simulink model "bObserver"  (R2020a)
settings: Solver=VariableStepAuto  StartTime=0.0  StopTime=1.5  FixedStep=0.0005  EnableMultiTasking=on
InitFcn:
  | kp=0.01;
  | ki=0.01;
  | 
  | k=2;
  | em=100000000;
  | GE=1/em;
  | GU=k*ki/GE;
  | GCE=k*kp/GU;
model workspace (MAT data in the model file):
  time = 0.8
values from neighbouring files (symbols this model uses):
  A1 = obj.boostConverter.A1    [BoostController.m]    (also in BoostConverter.m = [-obj.R/obj.L 0;0 -1/(obj.Ro*obj.C)]; BuckBoostConverter.m = [-obj.R/obj.L 0;0 -1/(obj.Ro*obj.C)]; obsmc.m = Asigma{1,1}; workspace_atual.mat = [-16.4  0; 0  -3.50877192982])
  A2 = obj.boostConverter.A2    [BoostController.m]    (also in BoostConverter.m = [-obj.R/obj.L -1/obj.L;1/obj.C -1/(obj.Ro*obj.C)]; BuckBoostConverter.m = [-obj.R/obj.L 1/obj.L;-1/obj.C -1/(obj.Ro*obj.C)]; obsmc.m = Asigma{1,2}; workspace_atual.mat = [-16.4  -200; 350.877192982  -3.50877192982])
  AlarmDeadTime = 0.50    (= 0.5)    [BoostFaultSimulation.m]    (also in workspace_atual.mat; workspace_certo.mat)
  B1 = obj.boostConverter.B1    [BoostController.m]    (also in BoostConverter.m = [1/obj.L;0]; BuckBoostConverter.m = [1/obj.L;0]; obsmc.m = Bsigma{1,1}; workspace_atual.mat = [200 0])
  B1f = [200 0]    [workspace_atual.mat]    (also in workspace_certo.mat)
  B2 = obj.boostConverter.B2    [BoostController.m]    (also in BoostConverter.m = obj.B1; obsmc.m = Bsigma{1,2}; workspace_atual.mat = [200 0]; workspace_certo.mat = [200 0])
  B2f = [200 0]    [workspace_atual.mat]    (also in workspace_certo.mat)
  boost_Amatrices = cat(3,obj.A1,obj.A2)    [BoostConverter.m]    (also in BuckBoostConverter.m; boostResults2Latex.m = boost.A_matrices(); workspace_atual.mat = [-16.4 0 0 -3.50877192982 -16.4 350.877192982 -200 -3.508771; workspace_certo.mat = [-16.4 0 0 -3.50877192982 -16.4 350.877192982 -200 -3.508771)
  boost_parameters = [obj.Ro,obj.R,obj.L,obj.C,obj.u]'    [BoostConverter.m]    (also in BuckBoostConverter.m; boostResults2Latex.m = boost.parameters(); workspace_atual.mat = [100 0.082 0.005 0.00285 190]; workspace_certo.mat = [100 0.082 0.005 0.00285 190])
  C = 1e-3    (= 0.001)    [boostResults2Latex.m]
  CiL = [0 1]    [workspace_atual.mat]    (also in workspace_certo.mat)
  Cmatrix = [1  0; 0  1]    [workspace_atual.mat]    (also in workspace_certo.mat)
  CVc = [1 0]    [workspace_atual.mat]    (also in workspace_certo.mat)
  D1 = [1  0; 0  1]    [workspace_atual.mat]    (also in workspace_certo.mat)
  F_11 = -16.4    [workspace_atual.mat]    (also in workspace_certo.mat)
  F_12 = -4812476.87956    [workspace_atual.mat]    (also in workspace_certo.mat)
  F_21 = -3.50877192982    [workspace_atual.mat]    (also in workspace_certo.mat)
  F_22 = -2.00703596657    [workspace_atual.mat]    (also in workspace_certo.mat)
  FaultClass = 0    [BoostFaultSimulation.m]    (also in workspace_atual.mat = 1; workspace_certo.mat = 1)
  H_1 = 13715.5123667    [workspace_atual.mat]    (also in workspace_certo.mat)
  iLFaultSwitch = 0    [BoostFaultSimulation.m]    (also in workspace_atual.mat; workspace_certo.mat)
  iLFaultTime = 1.70    (= 1.7)    [BoostFaultSimulation.m]    (also in workspace_atual.mat; workspace_certo.mat)
  iLGainFaultFactor = 15    [BoostFaultSimulation.m]    (also in workspace_atual.mat; workspace_certo.mat)
  iLNoiseFaultSwitch = 0    [BoostFaultSimulation.m]    (also in workspace_atual.mat; workspace_certo.mat)
  iLNoiseTime = 1.70    (= 1.7)    [BoostFaultSimulation.m]    (also in workspace_atual.mat; workspace_certo.mat)
  Jth = 2000    [workspace_atual.mat]    (also in workspace_certo.mat)
  L = 1e-3    (= 0.001)    [boostResults2Latex.m]    (also in obsmc.m = sdpvar(3,1,'full'))
  L_11 = -176809.798019    [workspace_atual.mat]    (also in workspace_certo.mat)
  L_12 = -66005538231.6    [workspace_atual.mat]    (also in workspace_certo.mat)
  L_21 = 0.0967961040176    [workspace_atual.mat]    (also in workspace_certo.mat)
  L_22 = 350.985265141    [workspace_atual.mat]    (also in workspace_certo.mat)
  LoadAddSignalSwitch = 1    [BoostFaultSimulation.m]    (also in workspace_atual.mat; workspace_certo.mat)
  LoadAddSwitch = 0    [BoostFaultSimulation.m]    (also in workspace_atual.mat; workspace_certo.mat)
  LoadAddTime = 0.90    (= 0.9)    [BoostFaultSimulation.m]    (also in workspace_atual.mat; workspace_certo.mat)
  LoadRemoveSignalSwitch = 1    [BoostFaultSimulation.m]    (also in workspace_atual.mat; workspace_certo.mat)
  LoadRemoveSwitch = 0    [BoostFaultSimulation.m]    (also in workspace_atual.mat; workspace_certo.mat)
  LoadRemoveTime = 0.90    (= 0.9)    [BoostFaultSimulation.m]    (also in workspace_atual.mat; workspace_certo.mat)
  LobsiL = [1737913.15707 66180.0912281]    [workspace_atual.mat]    (also in workspace_certo.mat)
  LobsVc = [61200 1]    [workspace_atual.mat]    (also in workspace_certo.mat)
  ObsEp = 70    [workspace_atual.mat]    (also in workspace_certo.mat)
  P = value(P)    [BoostController.m]    (also in boostResults2Latex.m = boost.calculateP(); obsmc.m = blkdiag(1/deltaAtilde(1,2),-1/deltaAtilde(2,1),1); workspace_atual.mat = [0.00235275094895  5.25738510027e-05; 5.25738510027e-05  0.0; workspace_certo.mat = [0.00235275094893  5.25738512446e-05; 5.25738512446e-05  0.0)
  Q_1 = [13715.5123667  1; 1  0]    [workspace_atual.mat]    (also in workspace_certo.mat)
  Q_2 = [1  0; 0.00750867981628  1]    [workspace_atual.mat]    (also in workspace_certo.mat)
  R = 0.1    [boostResults2Latex.m]    (also in workspace_atual.mat = 0.082; workspace_certo.mat = 0.082)
  ReconfigSwitch = 0    [BoostFaultSimulation.m]    (also in workspace_atual.mat; workspace_certo.mat)
  ReconfigTime = 1.707    [BoostFaultSimulation.m]    (also in workspace_atual.mat; workspace_certo.mat)
  rho = 5    [workspace_atual.mat]    (also in workspace_certo.mat)
  RMSfrequency = 47.61    [BoostFaultSimulation.m]    (also in workspace_atual.mat; workspace_certo.mat)
  Ro = 100    [BoostFaultSimulation.m]    (also in boostResults2Latex.m = 10; workspace_atual.mat; workspace_certo.mat)
  Smep = 80    [workspace_atual.mat]    (also in workspace_certo.mat)
  SourceAddSignalSwitch = 1    [BoostFaultSimulation.m]    (also in workspace_atual.mat; workspace_certo.mat)
  SourceAddSwitch = 0    [BoostFaultSimulation.m]    (also in workspace_atual.mat; workspace_certo.mat)
  SourceAddTime = 0.90    (= 0.9)    [BoostFaultSimulation.m]    (also in workspace_atual.mat; workspace_certo.mat)
  SourceAddVoltage = obj.SourceAddFactor*obj.u    [BoostFaultSimulation.m]    (also in workspace_atual.mat = 19; workspace_certo.mat = 19)
  SourceRemoveSignalSwitch = 1    [BoostFaultSimulation.m]    (also in workspace_atual.mat; workspace_certo.mat)
  SourceRemoveSwitch = 0    [BoostFaultSimulation.m]    (also in workspace_atual.mat; workspace_certo.mat)
  SourceRemoveTime = 0.90    (= 0.9)    [BoostFaultSimulation.m]    (also in workspace_atual.mat; workspace_certo.mat)
  SourceRemoveVoltage = obj.SourceRemoveFactor*obj.u    [BoostFaultSimulation.m]    (also in workspace_atual.mat = 19; workspace_certo.mat = 19)
  T_1 = [1 -13715.5123667]    [workspace_atual.mat]    (also in workspace_certo.mat)
  T_2 = [-0.00750867981628 1]    [workspace_atual.mat]    (also in workspace_certo.mat)
  ueq = 0.5    [workspace_atual.mat]    (also in workspace_certo.mat)
  uf = 190    [workspace_atual.mat]    (also in workspace_certo.mat)
  VcFaultSwitch = 0    [BoostFaultSimulation.m]    (also in workspace_atual.mat; workspace_certo.mat)
  VcFaultTime = 1.70    (= 1.7)    [BoostFaultSimulation.m]    (also in workspace_atual.mat; workspace_certo.mat)
  VcGainFaultFactor = 15    [BoostFaultSimulation.m]    (also in workspace_atual.mat; workspace_certo.mat)
  VcNoiseFaultSwitch = 0    [BoostFaultSimulation.m]    (also in workspace_atual.mat; workspace_certo.mat)
  VcNoiseTime = 1.70    (= 1.7)    [BoostFaultSimulation.m]    (also in workspace_atual.mat; workspace_certo.mat)
  ve = 380    [BoostFaultSimulation.m]    (also in boostResults2Latex.m = 100; workspace_atual.mat; workspace_certo.mat)
  x_e = [ie;ve]    [BoostConverter.m]    (also in BuckBoostConverter.m)
  xe = obj.boostConverter.equilibriumstate(ve)    [BoostController.m]    (also in workspace_atual.mat = [7.62509288104 380]; workspace_certo.mat = [7.62509288104 380])
undefined symbols (not defined in the file or in its folder): Atilde1, Atilde2, B1u, Ctilde1, Dtilde1, Dtilde2, F, F1, G, G1, MAXnet, MINnet
libraries: neural x36, powerlib x34, dspstat3 x11, PhdLibrary x10, simulink x7, dspmtrx3 x6, powerlib_meascontrol x4, dspmathops x4
(part 6 of 6)

== system bObserver/ROSLSO/Fault Diagnostics/Fault Identification Neural Netowrk/Pattern Recognition Neural Network1/Layer 1/IW{1,1} ==
  "pd{1,1}" : Inport  PortDimensions=3
      mask Display: e = 0.06;c1 = [120 230 180]/255;c2 = ([120 230 180]+0)/(256+128);c3 = ([120 230 180]+128)/(256+128);patch([0 1 1 0],[0 0 1 1],c1);patch([0 1 1 1-e 1-e 0+e],[0 0 1 1-e 0+e 0+e],c2);patch([0 0 1 1-e 0+e 0+e],[0 1 1 1-e 1-e 0+e],c3);plot([0 1 1 0 0],[0 0 1 1 0]);
  "IW{1,1}(1,:)'" : Constant  Value=[1.4620077904292643200534485004027374088764190673828125;1.1479316995695467706894987713894806802272796630859375;-0.75309198928315967958013743555056862533092498779296875]
      mask Display: e = 0.06;c1 = [120 150 230]/255;c2 = ([120 150 230]+0)/383;c3 = ([120 150 230]+128)/383;patch([0 1 1 0],[0 0 1 1],c1);patch([0 1 1 1-e 1-e 0+e],[0 0 1 1-e 0+e 0+e],c2);patch([0 0 1 1-e 0+e 0+e],[0 1 1 1-e 1-e 0+e],c3);plot([0 1 1 0 0],[0 0 1 1 0]);disp('Weights');
  "IW{1,1}(2,:)'" : Constant  Value=[-4.88697839849253856669974993565119802951812744140625;-8.405003124593715568835250451229512691497802734375;5.794020912154170588337365188635885715484619140625]
      mask Display: e = 0.06;c1 = [120 150 230]/255;c2 = ([120 150 230]+0)/383;c3 = ([120 150 230]+128)/383;patch([0 1 1 0],[0 0 1 1],c1);patch([0 1 1 1-e 1-e 0+e],[0 0 1 1-e 0+e 0+e],c2);patch([0 0 1 1-e 0+e 0+e],[0 1 1 1-e 1-e 0+e],c3);plot([0 1 1 0 0],[0 0 1 1 0]);disp('Weights');
  "IW{1,1}(3,:)'" : Constant  Value=[14.0491237632533483292718301527202129364013671875;1.08719679537565827587286548805423080921173095703125;21.342540048378236150483644451014697551727294921875]
      mask Display: e = 0.06;c1 = [120 150 230]/255;c2 = ([120 150 230]+0)/383;c3 = ([120 150 230]+128)/383;patch([0 1 1 0],[0 0 1 1],c1);patch([0 1 1 1-e 1-e 0+e],[0 0 1 1-e 0+e 0+e],c2);patch([0 0 1 1-e 0+e 0+e],[0 1 1 1-e 1-e 0+e],c3);plot([0 1 1 0 0],[0 0 1 1 0]);disp('Weights');
  "IW{1,1}(4,:)'" : Constant  Value=[-16.064558456108986916888170526362955570220947265625;9.3944940835869257256263153976760804653167724609375;10.4677174695698536055488148122094571590423583984375]
      mask Display: e = 0.06;c1 = [120 150 230]/255;c2 = ([120 150 230]+0)/383;c3 = ([120 150 230]+128)/383;patch([0 1 1 0],[0 0 1 1],c1);patch([0 1 1 1-e 1-e 0+e],[0 0 1 1-e 0+e 0+e],c2);patch([0 0 1 1-e 0+e 0+e],[0 1 1 1-e 1-e 0+e],c3);plot([0 1 1 0 0],[0 0 1 1 0]);disp('Weights');
  Mux : Mux
      mask Display: e = 0.06;c1 = [120 150 230]/255;c2 = ([120 150 230]+0)/383;c3 = ([120 150 230]+128)/383;patch([0 1 1 0],[0 0 1 1],c1);patch([0 1 1 1-e 1-e 0+e],[0 0 1 1-e 0+e 0+e],c2);patch([0 0 1 1-e 0+e 0+e],[0 1 1 1-e 1-e 0+e],c3);plot([0 1 1 0 0],[0 0 1 1 0]);disp('Mux');
  dotprod{1..4} (4 alike) : neural/Weight Functions/dotprod
  "iz{1,1}" : Outport
      mask Display: e = 0.06;c1 = [120 230 180]/255;c2 = ([120 230 180]+0)/(256+128);c3 = ([120 230 180]+128)/(256+128);patch([0 1 1 0],[0 0 1 1],c1);patch([0 1 1 1-e 1-e 0+e],[0 0 1 1-e 0+e 0+e],c2);patch([0 0 1 1-e 0+e 0+e],[0 1 1 1-e 1-e 0+e],c3);plot([0 1 1 0 0],[0 0 1 1 0]);
  wires:
  "IW{1,1}(1,:)'"/1 -> dotprod1/1
  "pd{1,1}"/1 -> dotprod1/2, dotprod2/2, dotprod3/2, dotprod4/2
  dotprod1/1 -> Mux/1
  "IW{1,1}(2,:)'"/1 -> dotprod2/1
  dotprod2/1 -> Mux/2
  "IW{1,1}(3,:)'"/1 -> dotprod3/1
  dotprod3/1 -> Mux/3
  "IW{1,1}(4,:)'"/1 -> dotprod4/1
  dotprod4/1 -> Mux/4
  Mux/1 -> "iz{1,1}"/1

== system bObserver/ROSLSO/Fault Diagnostics/Fault Identification Neural Netowrk/Pattern Recognition Neural Network1/Layer 2/Delays 1 ==
  "p{2}" : Inport  PortDimensions=4
      mask Display: e = 0.06;c1 = [120 230 180]/255;c2 = ([120 230 180]+0)/(256+128);c3 = ([120 230 180]+128)/(256+128);patch([0 1 1 0],[0 0 1 1],c1);patch([0 1 1 1-e 1-e 0+e],[0 0 1 1-e 0+e 0+e],c2);patch([0 0 1 1-e 0+e 0+e],[0 1 1 1-e 1-e 0+e],c3);plot([0 1 1 0 0],[0 0 1 1 0]);
  mux : Mux  Inputs=1
      mask Display: e = 0.06;c1 = [120 150 230]/255;c2 = ([120 150 230]+0)/383;c3 = ([120 150 230]+128)/383;patch([0 1 1 0],[0 0 1 1],c1);patch([0 1 1 1-e 1-e 0+e],[0 0 1 1-e 0+e 0+e],c2);patch([0 0 1 1-e 0+e 0+e],[0 1 1 1-e 1-e 0+e],c3);plot([0 1 1 0 0],[0 0 1 1 0]);disp('Mux')
  "pd{2,1}" : Outport
      mask Display: e = 0.06;c1 = [120 230 180]/255;c2 = ([120 230 180]+0)/(256+128);c3 = ([120 230 180]+128)/(256+128);patch([0 1 1 0],[0 0 1 1],c1);patch([0 1 1 1-e 1-e 0+e],[0 0 1 1-e 0+e 0+e],c2);patch([0 0 1 1-e 0+e 0+e],[0 1 1 1-e 1-e 0+e],c3);plot([0 1 1 0 0],[0 0 1 1 0]);
  wires:
  "p{2}"/1 -> mux/1
  mux/1 -> "pd{2,1}"/1

== system bObserver/ROSLSO/Fault Diagnostics/Fault Identification Neural Netowrk/Pattern Recognition Neural Network1/Layer 2/LW{2,1} ==
  "ad{2,1}" : Inport  PortDimensions=4
      mask Display: e = 0.06;c1 = [120 230 180]/255;c2 = ([120 230 180]+0)/(256+128);c3 = ([120 230 180]+128)/(256+128);patch([0 1 1 0],[0 0 1 1],c1);patch([0 1 1 1-e 1-e 0+e],[0 0 1 1-e 0+e 0+e],c2);patch([0 0 1 1-e 0+e 0+e],[0 1 1 1-e 1-e 0+e],c3);plot([0 1 1 0 0],[0 0 1 1 0]);
  "IW{2,1}(1,:)'" : Constant  Value=[1.904651848873672559392389302956871688365936279296875;-0.84465724683745302403536925339722074568271636962890625;-3.4679025925519777473482463392429053783416748046875;11.422204742389372000843650312162935733795166015625]
      mask Display: e = 0.06;c1 = [120 150 230]/255;c2 = ([120 150 230]+0)/383;c3 = ([120 150 230]+128)/383;patch([0 1 1 0],[0 0 1 1],c1);patch([0 1 1 1-e 1-e 0+e],[0 0 1 1-e 0+e 0+e],c2);patch([0 0 1 1-e 0+e 0+e],[0 1 1 1-e 1-e 0+e],c3);plot([0 1 1 0 0],[0 0 1 1 0]);disp('weights');
  "IW{2,1}(2,:)'" : Constant  Value=[5.437015296800307595503909396938979625701904296875;9.1687061761547976601605114410631358623504638671875;23.548730693488327148088501417078077793121337890625;9.759995330560929716057216865010559558868408203125]
      mask Display: e = 0.06;c1 = [120 150 230]/255;c2 = ([120 150 230]+0)/383;c3 = ([120 150 230]+128)/383;patch([0 1 1 0],[0 0 1 1],c1);patch([0 1 1 1-e 1-e 0+e],[0 0 1 1-e 0+e 0+e],c2);patch([0 0 1 1-e 0+e 0+e],[0 1 1 1-e 1-e 0+e],c3);plot([0 1 1 0 0],[0 0 1 1 0]);disp('weights');
  "IW{2,1}(3,:)'" : Constant  Value=[-7.4815615461727844603956327773630619049072265625;-8.028817388537188293184954090975224971771240234375;-11.2939495357742867298611599835567176342010498046875;-9.9286767851498662906806202954612672328948974609375]
      mask Display: e = 0.06;c1 = [120 150 230]/255;c2 = ([120 150 230]+0)/383;c3 = ([120 150 230]+128)/383;patch([0 1 1 0],[0 0 1 1],c1);patch([0 1 1 1-e 1-e 0+e],[0 0 1 1-e 0+e 0+e],c2);patch([0 0 1 1-e 0+e 0+e],[0 1 1 1-e 1-e 0+e],c3);plot([0 1 1 0 0],[0 0 1 1 0]);disp('weights');
  "IW{2,1}(4,:)'" : Constant  Value=[-0.9996034096479060604423239055904559791088104248046875;10.7127959018867926488383091054856777191162109375;-15.9786358721355643552897163317538797855377197265625;-16.727505534885494853369891643524169921875]
      mask Display: e = 0.06;c1 = [120 150 230]/255;c2 = ([120 150 230]+0)/383;c3 = ([120 150 230]+128)/383;patch([0 1 1 0],[0 0 1 1],c1);patch([0 1 1 1-e 1-e 0+e],[0 0 1 1-e 0+e 0+e],c2);patch([0 0 1 1-e 0+e 0+e],[0 1 1 1-e 1-e 0+e],c3);plot([0 1 1 0 0],[0 0 1 1 0]);disp('weights');
  "IW{2,1}(5,:)'" : Constant  Value=[1.6498552634234948666147602125420235097408294677734375;-11.401380066045131655982913798652589321136474609375;7.07176418368389203550350430305115878582000732421875;5.3013653852550621792261154041625559329986572265625]
      mask Display: e = 0.06;c1 = [120 150 230]/255;c2 = ([120 150 230]+0)/383;c3 = ([120 150 230]+128)/383;patch([0 1 1 0],[0 0 1 1],c1);patch([0 1 1 1-e 1-e 0+e],[0 0 1 1-e 0+e 0+e],c2);patch([0 0 1 1-e 0+e 0+e],[0 1 1 1-e 1-e 0+e],c3);plot([0 1 1 0 0],[0 0 1 1 0]);disp('weights');
  Mux : Mux  Inputs=5
      mask Display: e = 0.06;c1 = [120 150 230]/255;c2 = ([120 150 230]+0)/383;c3 = ([120 150 230]+128)/383;patch([0 1 1 0],[0 0 1 1],c1);patch([0 1 1 1-e 1-e 0+e],[0 0 1 1-e 0+e 0+e],c2);patch([0 0 1 1-e 0+e 0+e],[0 1 1 1-e 1-e 0+e],c3);plot([0 1 1 0 0],[0 0 1 1 0]);disp('Mux');
  dotprod{1..5} (5 alike) : neural/Weight Functions/dotprod
  "lz{2,1}" : Outport
      mask Display: e = 0.06;c1 = [120 230 180]/255;c2 = ([120 230 180]+0)/(256+128);c3 = ([120 230 180]+128)/(256+128);patch([0 1 1 0],[0 0 1 1],c1);patch([0 1 1 1-e 1-e 0+e],[0 0 1 1-e 0+e 0+e],c2);patch([0 0 1 1-e 0+e 0+e],[0 1 1 1-e 1-e 0+e],c3);plot([0 1 1 0 0],[0 0 1 1 0]);
  wires:
  "IW{2,1}(1,:)'"/1 -> dotprod1/1
  "ad{2,1}"/1 -> dotprod1/2, dotprod2/2, dotprod3/2, dotprod4/2, dotprod5/2
  dotprod1/1 -> Mux/1
  "IW{2,1}(2,:)'"/1 -> dotprod2/1
  dotprod2/1 -> Mux/2
  "IW{2,1}(3,:)'"/1 -> dotprod3/1
  dotprod3/1 -> Mux/3
  "IW{2,1}(4,:)'"/1 -> dotprod4/1
  dotprod4/1 -> Mux/4
  "IW{2,1}(5,:)'"/1 -> dotprod5/1
  dotprod5/1 -> Mux/5
  Mux/1 -> "lz{2,1}"/1

== matlab function bObserver/ROSLSO/Chaveado_fixo1/Controlador Chavead/MatirxControle/control_law  ==
  data: x_e input; sigma output; P input; boost_Amatrices input; x input; control_matrix output
function [sigma, control_matrix] = fcn(x_e, P, boost_Amatrices, x)
 
A1 = boost_Amatrices(:,:,1);
A2 = boost_Amatrices(:,:,2);

control_matrix = P*((A1 - A2)*x_e);
 
if control_matrix'*(x-x_e) <= 0
    sigma = 1;%1
else
    sigma = 0; %2
end

== matlab function bObserver/ROSLSO/Chaveado_fixo1/Controlador Chavead/MatirxControle/xe ==
  data: i_e output; boost_parameters input; ve input; x_e output
function [i_e,x_e] = fcn(boost_parameters,ve)
%parameters = (Ro,R,L,C,u)
%     
Ro = boost_parameters(1);
R = boost_parameters(2);
u = boost_parameters(5);

delta_ie = (-u/R)^2 - (4*ve^2)/(R*Ro);
i_e = real(((u/R) - sqrt(complex(delta_ie)))/2);  

x_e = [i_e;ve];

== matlab function bObserver/ROSLSO/Controlador1/xe ==
  data: boost_parameters input; ve input; x_e output; i_e output
function [x_e,i_e] = fcn(boost_parameters,ve)
%parameters = (Ro,R,L,C,u)
%     
R = boost_parameters(2);
Ro = boost_parameters(1);
u = boost_parameters(5);

delta_ie = (-u/R)^2 - (4*ve^2)/(R*Ro);
i_e = real(((u/R) - sqrt(complex(delta_ie)))/2);  
x_e = [i_e;ve];

== matlab function bObserver/Slding Mode/Controlador1/xe ==
  data: boost_parameters input; ve input; x_e output; i_e output
function [x_e,i_e] = fcn(boost_parameters,ve)
%parameters = (Ro,R,L,C,u)
%     
R = boost_parameters(2);
Ro = boost_parameters(1);
u = boost_parameters(5);

delta_ie = (-u/R)^2 - (4*ve^2)/(R*Ro);
i_e = real(((u/R) - sqrt(complex(delta_ie)))/2);  
x_e = [i_e;ve];
